simulink model "test_com_PowerLimitation_adaptTorquePart"  (R2017a)
settings: Solver=FixedStepDiscrete  StartTime=0.0  StopTime=160  RelTol=1e-3
libraries: simulink x1
settings Model: Creator=gt_testing  LastModifiedBy=rieth

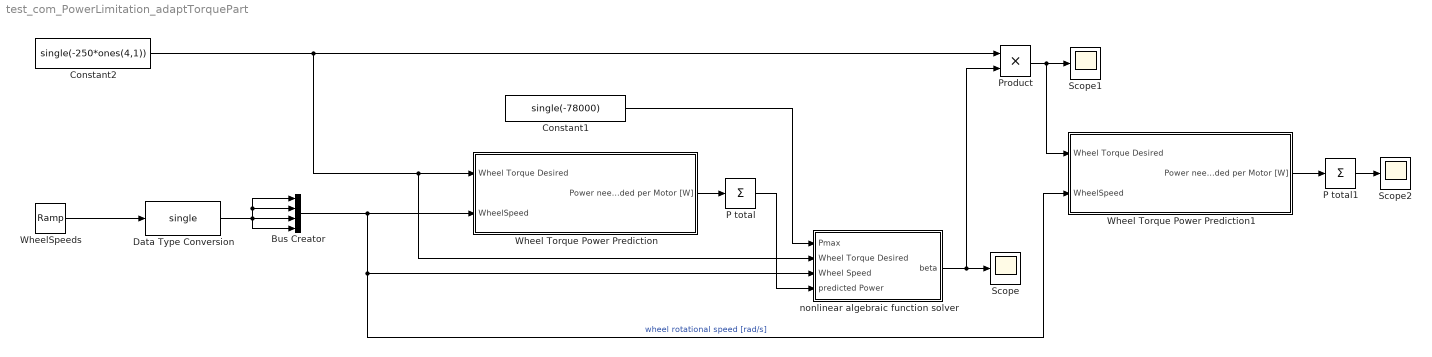
== system test_com_PowerLimitation_adaptTorquePart ==
  Bus Creator : BusCreator  Inputs=4
  Constant1 : Constant  Value=single(-78000)
  Constant2 : Constant  Value=single(-250*ones(4,1))  SampleTime=0.001
  Data Type Conversion : DataTypeConversion  OutDataTypeStr=single
  P total : Sum  Inputs=+
  P total1 : Sum  Inputs=+
  Product : Product
  Scope : Scope
  Scope1 : Scope
  Scope2 : Scope
  Wheel Torque Power Prediction : Subsystem
  Wheel Torque Power Prediction1 : Subsystem
  WheelSpeeds : simulink/Sources/Ramp  slope=-1  start=1  X0=151
  nonlinear algebraic function solver : Subsystem
  wires:
  nonlinear algebraic function solver/1(beta) -> Scope/1, Product/2
  Wheel Torque Power Prediction/1(Power needed per Motor [W]) -> P total/1
  P total/1 -> nonlinear algebraic function solver/4(predicted Power)
  Constant2/1 -> nonlinear algebraic function solver/2(Wheel Torque Desired), Wheel Torque Power Prediction/1(Wheel Torque Desired), Product/1
  Constant1/1 -> nonlinear algebraic function solver/1(Pmax)
  Bus Creator/1 -> nonlinear algebraic function solver/3(Wheel Speed), Wheel Torque Power Prediction1/2(WheelSpeed), Wheel Torque Power Prediction/2(WheelSpeed)  "wheel rotational speed [rad/s]"
  WheelSpeeds/1 -> Data Type Conversion/1
  Data Type Conversion/1 -> Bus Creator/2, Bus Creator/1, Bus Creator/4, Bus Creator/3
  Product/1 -> Scope1/1, Wheel Torque Power Prediction1/1(Wheel Torque Desired)
  Wheel Torque Power Prediction1/1(Power needed per Motor [W]) -> P total1/1
  P total1/1 -> Scope2/1

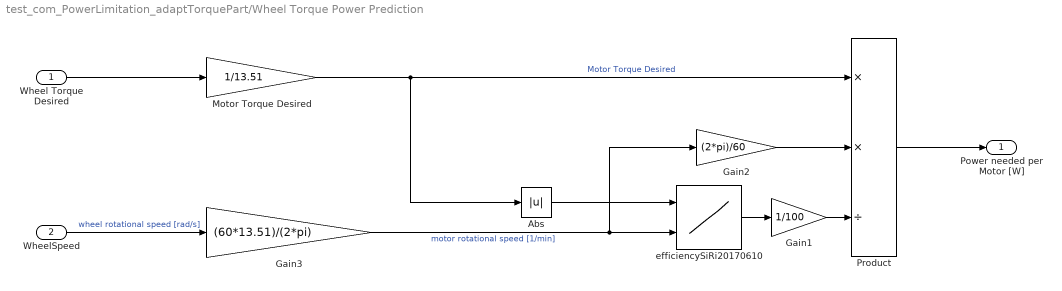
== system test_com_PowerLimitation_adaptTorquePart/Wheel Torque Power Prediction ==
  Wheel Torque Desired : Inport
  WheelSpeed : Inport  Port=2
  Abs : Abs
  Gain1 : Gain  Gain=1/100
  Gain2 : Gain  Gain=(2*pi)/60
  Gain3 : Gain  Gain=(60*13.51)/(2*pi)
  Motor Torque Desired : Gain  Gain=1/13.51
  Product : Product  Inputs=**/
  efficiencySiRi20170610 : Lookup_n-D  BreakpointsForDimension1=single([1,3.2,3.9,8.7,10,11.3,16.2,20.3,24,26.9,28.3]);  BreakpointsForDimension2=single([48,1960,3950,5880,7870,9840,11780,13740,14720,15710,17690,19640]);  Table="single( reshape( [94 93 92 91 90 90 90 90 90 90 90 90; 99.36774129\t90.61029352\t90.48980391\t90.9585099\t91.97303205\t86.66621940\t86.45154548\t89.45556778\t93.49708755\t90.20622767\t96.32187851\t93.77483204; 31.27753348\t89.58805789\t90.35051471\t91.0088400\t91.34257504\t92.79112863\t93.43970070\t92.86254617\t95.49044846\t91.88713991\t92.09660288\t99.38740423; 31.22057366\t88.54516887\t91.41259271\t91.9339048\t92.80185490\t93.37850287\t93.37968650\t93.43660779\t95.56974312\t93.62737163\t98.23400855\t97.68028598;  19.06082130\t88.16649558\t92.11595977\t92.90571858\t94.06474181\t93.59829873\t93.68368928\t93.99821230\t94.48495482\t93.64934183\t97.64599471\t99.79304925; 22.65493310\t85.04354735\t90.63432599\t90.89186387\t93.01206035\t92.42222619\t93.04151248\t93.12674620\t94.62498470\t93.19873407\t97.48235007\t99.63288088; 14.35381991\t81.97479573\t88.38188275\t90.58879348\t91.42237266\t91.86404458\t91.96724861\t92.60660720\t93.61744476\t92.73660389\t96.28617258\t97.91800590; 9.871996419\t75.78855723\t84.58478190\t87.19329262\t89.29452440\t90.10911954\t88.99885889\t91.24022984\t92.50845489\t92.30525632\t92.70068550\t95.95176799; 7.166365164\t66.33041277\t78.12603510\t81.72006745\t85.16747699\t86.66493509\t87.05734065\t89.50257798\t89.70411810\t90.50722583 90.50722583 90.50722583; 5.521446362\t64.00758121\t75.81765563\t81.30737314\t85.24988669\t87.40396493 87.40396493 87.40396493 87.40396493 87.40396493 87.40396493 87.40396493; 4.758428457\t61.91902319\t74.24685691\t80.55482871\t83.61528364\t85.08425625 85.08425625 85.08425625 85.08425625 85.08425625 85.08425625 85.08425625], 11, 12 ) );"  InternalRulePriority=Speed  RndMeth=Simplest  InputSameDT=on
  Power needed per Motor [W] : Outport  OutDataTypeStr=single
  wires:
  Wheel Torque Desired/1 -> Motor Torque Desired/1
  Motor Torque Desired/1 -> Product/1, Abs/1  "Motor Torque Desired"
  Product/1 -> Power needed per Motor [W]/1
  Abs/1 -> efficiencySiRi20170610/1
  Gain1/1 -> Product/3
  efficiencySiRi20170610/1 -> Gain1/1
  WheelSpeed/1 -> Gain3/1  "wheel rotational speed [rad/s]"
  Gain3/1 -> Gain2/1, efficiencySiRi20170610/2  "motor rotational speed [1/min]"
  Gain2/1 -> Product/2

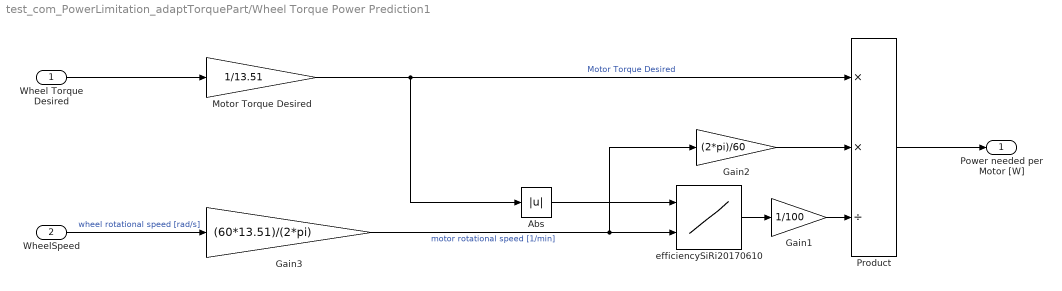
== system test_com_PowerLimitation_adaptTorquePart/Wheel Torque Power Prediction1 ==
  Wheel Torque Desired : Inport
  WheelSpeed : Inport  Port=2
  Abs : Abs
  Gain1 : Gain  Gain=1/100
  Gain2 : Gain  Gain=(2*pi)/60
  Gain3 : Gain  Gain=(60*13.51)/(2*pi)
  Motor Torque Desired : Gain  Gain=1/13.51
  Product : Product  Inputs=**/
  efficiencySiRi20170610 : Lookup_n-D  BreakpointsForDimension1=single([1,3.2,3.9,8.7,10,11.3,16.2,20.3,24,26.9,28.3]);  BreakpointsForDimension2=single([48,1960,3950,5880,7870,9840,11780,13740,14720,15710,17690,19640]);  Table="single( reshape( [94 93 92 91 90 90 90 90 90 90 90 90; 99.36774129\t90.61029352\t90.48980391\t90.9585099\t91.97303205\t86.66621940\t86.45154548\t89.45556778\t93.49708755\t90.20622767\t96.32187851\t93.77483204; 31.27753348\t89.58805789\t90.35051471\t91.0088400\t91.34257504\t92.79112863\t93.43970070\t92.86254617\t95.49044846\t91.88713991\t92.09660288\t99.38740423; 31.22057366\t88.54516887\t91.41259271\t91.9339048\t92.80185490\t93.37850287\t93.37968650\t93.43660779\t95.56974312\t93.62737163\t98.23400855\t97.68028598;  19.06082130\t88.16649558\t92.11595977\t92.90571858\t94.06474181\t93.59829873\t93.68368928\t93.99821230\t94.48495482\t93.64934183\t97.64599471\t99.79304925; 22.65493310\t85.04354735\t90.63432599\t90.89186387\t93.01206035\t92.42222619\t93.04151248\t93.12674620\t94.62498470\t93.19873407\t97.48235007\t99.63288088; 14.35381991\t81.97479573\t88.38188275\t90.58879348\t91.42237266\t91.86404458\t91.96724861\t92.60660720\t93.61744476\t92.73660389\t96.28617258\t97.91800590; 9.871996419\t75.78855723\t84.58478190\t87.19329262\t89.29452440\t90.10911954\t88.99885889\t91.24022984\t92.50845489\t92.30525632\t92.70068550\t95.95176799; 7.166365164\t66.33041277\t78.12603510\t81.72006745\t85.16747699\t86.66493509\t87.05734065\t89.50257798\t89.70411810\t90.50722583 90.50722583 90.50722583; 5.521446362\t64.00758121\t75.81765563\t81.30737314\t85.24988669\t87.40396493 87.40396493 87.40396493 87.40396493 87.40396493 87.40396493 87.40396493; 4.758428457\t61.91902319\t74.24685691\t80.55482871\t83.61528364\t85.08425625 85.08425625 85.08425625 85.08425625 85.08425625 85.08425625 85.08425625], 11, 12 ) );"  InternalRulePriority=Speed  RndMeth=Simplest  InputSameDT=on
  Power needed per Motor [W] : Outport  OutDataTypeStr=single
  wires:
  Gain2/1 -> Product/2
  Gain3/1 -> efficiencySiRi20170610/2, Gain2/1  "motor rotational speed [1/min]"
  WheelSpeed/1 -> Gain3/1  "wheel rotational speed [rad/s]"
  efficiencySiRi20170610/1 -> Gain1/1
  Gain1/1 -> Product/3
  Abs/1 -> efficiencySiRi20170610/1
  Product/1 -> Power needed per Motor [W]/1
  Motor Torque Desired/1 -> Abs/1, Product/1  "Motor Torque Desired"
  Wheel Torque Desired/1 -> Motor Torque Desired/1

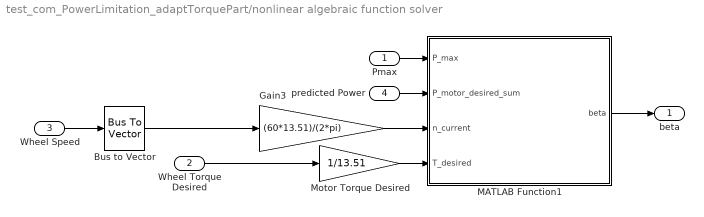
== system test_com_PowerLimitation_adaptTorquePart/nonlinear algebraic function solver ==
  Pmax : Inport
  Wheel Torque Desired : Inport  Port=2
  Wheel Speed : Inport  Port=3
  predicted Power : Inport  Port=4
  Bus to Vector : BusToVector
  Gain3 : Gain  Gain=(60*13.51)/(2*pi)
  MATLAB Function1 : MATLAB Function  TreatAsAtomicUnit=on
  Motor Torque Desired : Gain  Gain=1/13.51
  beta : Outport
  wires:
  MATLAB Function1/1(beta) -> beta/1
  Pmax/1 -> MATLAB Function1/1(P_max)
  Wheel Torque Desired/1 -> Motor Torque Desired/1
  Wheel Speed/1 -> Bus to Vector/1
  Motor Torque Desired/1 -> MATLAB Function1/4(T_desired)
  Bus to Vector/1 -> Gain3/1
  Gain3/1 -> MATLAB Function1/3(n_current)
  predicted Power/1 -> MATLAB Function1/2(P_motor_desired_sum)

== matlab function test_com_PowerLimitation_adaptTorquePart/nonlinear algebraic function solver/MATLAB Function1 ==
  data: P_max input single size=1; P_motor_desired_sum input single size=[1 1]; n_current input single size=[4,1]; T_desired input; beta output single size=1
function beta  = adaptTorque( P_max, P_motor_desired_sum, n_current,T_desired)

P_max = abs(P_max);
P_motor_desired_sum = abs(P_motor_desired_sum);
T_desired = abs(T_desired);

efficiency = zeros(4,1);
% efficiency_desired = zeros(4,1);

efficiency_complete = single( reshape( [94 93 92 91 90 90 90 90 90 90 90 90; ... 
                                        99.36774129	90.61029352	90.48980391	90.9585099	91.97303205	86.66621940	86.45154548	89.45556778	93.49708755	90.20622767	96.32187851	93.77483204; ...
                                        31.27753348	89.58805789	90.35051471	91.0088400	91.34257504	92.79112863	93.43970070	92.86254617	95.49044846	91.88713991	92.09660288	99.38740423; ...
                                        31.22057366	88.54516887	91.41259271	91.9339048	92.80185490	93.37850287	93.37968650	93.43660779	95.56974312	93.62737163	98.23400855	97.68028598; ...
                                        19.06082130	88.16649558	92.11595977	92.90571858	94.06474181	93.59829873	93.68368928	93.99821230	94.48495482	93.64934183	97.64599471	99.79304925; ...
                                        22.65493310	85.04354735	90.63432599	90.89186387	93.01206035	92.42222619	93.04151248	93.12674620	94.62498470	93.19873407	97.48235007	99.63288088; ...
                                        14.35381991	81.97479573	88.38188275	90.58879348	91.42237266	91.86404458	91.96724861	92.60660720	93.61744476	92.73660389	96.28617258	97.91800590; ...
                                        9.871996419	75.78855723	84.58478190	87.19329262	89.29452440	90.10911954	88.99885889	91.24022984	92.50845489	92.30525632	92.70068550	95.95176799; ...
                                        7.166365164	66.33041277	78.12603510	81.72006745	85.16747699	86.66493509	87.05734065	89.50257798	89.70411810	90.50722583 90.50722583 90.50722583; ...
                                        5.521446362	64.00758121	75.81765563	81.30737314	85.24988669	87.40396493 87.40396493 87.40396493 87.40396493 87.40396493 87.40396493 87.40396493; ...
                                        4.758428457	61.91902319	74.24685691	80.55482871	83.61528364	85.08425625 85.08425625 85.08425625 85.08425625 85.08425625 85.08425625 85.08425625], 11, 12 ) );
                         
T_complete = single([1,3.2,3.9,8.7,10,11.3,16.2,20.3,24,26.9,28.3]);
n_complete = single([48,1960,3950,5880,7870,9840,11780,13740,14720,15710,17690,19640]); 

n_current_radps = 2*pi/60 * n_current; %n_current in umdrehungen pro minute, umrechnung in rad pro sekunde 

% %Abfangen von out-of-range Werten
% for i = 1:4
%     if abs(T_desired(i)) > 28.3 
%         T_desired(i) = sign(T_desired(i))*single(28.3);
%     elseif T_desired(i) < 1
%         T_desired(i) = sign(T_desired(i))*single(1);
%     end
% end
% 
% efficiency_desired(1) = diag( interpn( T_complete, n_complete, efficiency_complete, abs(T_desired(1)), n_current(1), 'linear' ) ) / 100; %percentage
% efficiency_desired(2) = diag( interpn( T_complete, n_complete, efficiency_complete, abs(T_desired(2)), n_current(2), 'linear' ) ) / 100; %percentage
% efficiency_desired(3) = diag( interpn( T_complete, n_complete, efficiency_complete, abs(T_desired(3)), n_current(3), 'linear' ) ) / 100; %percentage
% efficiency_desired(4) = diag( interpn( T_complete, n_complete, efficiency_complete, abs(T_desired(4)), n_current(4), 'linear' ) ) / 100; %percentage
% 
% P_motor_desired_fl = T_desired(1)*n_current_radps(1)/efficiency_desired(1);
% P_motor_desired_fr = T_desired(2)*n_current_radps(2)/efficiency_desired(2);
% P_motor_desired_rl = T_desired(3)*n_current_radps(3)/efficiency_desired(3);
% P_motor_desired_rr = T_desired(4)*n_current_radps(4)/efficiency_desired(4);
% 
% P_motor_desired_sum = P_motor_desired_fl + P_motor_desired_fr + P_motor_desired_rl + P_motor_desired_rr;


% 
% if x < 0
%     x = single(0);
% elseif x > 1
%     x = single(1);
% end

T_adapted_old = T_desired + 1;
efficiency_old = single( zeros( 4, 1 ) );
T_adapted = T_desired;
P_Whatever = single( zeros( 4, 1 ) );
P_motor_adap_sum = P_motor_desired_sum;
condAdaptionCalculation = P_motor_adap_sum - P_max;

if condAdaptionCalculation > 0
    x = P_max/P_motor_desired_sum;
else
	x = single(1);
end

while condAdaptionCalculation > 0
    
    %Abfangen von out-of-range Werten
    for i = 1:4
        if abs(T_adapted(i)) > 28.3 
            T_adapted(i) = single(28.3);
        elseif T_adapted(i) < 1
            T_adapted(i) = single(1);
        end
    end
    
    % Berechnen des Wirkungsgrades mittels angepasstem Moment
    efficiency(1) = diag( interpn( T_complete, n_complete, efficiency_complete, T_adapted(1), n_current(1), 'linear' ) ) / 100; %percentage
    efficiency(2) = diag( interpn( T_complete, n_complete, efficiency_complete, T_adapted(2), n_current(2), 'linear' ) ) / 100; %percentage
    efficiency(3) = diag( interpn( T_complete, n_complete, efficiency_complete, T_adapted(3), n_current(3), 'linear' ) ) / 100; %percentage
    efficiency(4) = diag( interpn( T_complete, n_complete, efficiency_complete, T_adapted(4), n_current(4), 'linear' ) ) / 100; %percentage
        
    % Ableiten der Effizienz nach Korrekturfaktor
    DEfficiency_fl = ( efficiency(1) - efficiency_old(1) )./( T_adapted(1) - T_adapted_old(1) );
    DEfficiency_fr = ( efficiency(2) - efficiency_old(2) )./( T_adapted(2) - T_adapted_old(2) );
    DEfficiency_rl = ( efficiency(3) - efficiency_old(3) )./( T_adapted(3) - T_adapted_old(3) );
    DEfficiency_rr = ( efficiency(4) - efficiency_old(4) )./( T_adapted(4) - T_adapted_old(4) );
    DEfficiency = [DEfficiency_fl;DEfficiency_fr;DEfficiency_rl;DEfficiency_rr];
    
    % induced power 
    P_motor_ind_fl = T_adapted_old(1)*n_current_radps(1)/efficiency(1); 
    P_motor_ind_fr = T_adapted_old(2)*n_current_radps(2)/efficiency(2);
    P_motor_ind_rl = T_adapted_old(3)*n_current_radps(3)/efficiency(3);
    P_motor_ind_rr = T_adapted_old(4)*n_current_radps(4)/efficiency(4);    
    P_motor_ind = [P_motor_ind_fl;P_motor_ind_fr;P_motor_ind_rl;P_motor_ind_rr]; 
         
    % adapted induced power
    P_motor_adap_fl = T_adapted(1)*n_current_radps(1)/efficiency(1); 
    P_motor_adap_fr = T_adapted(2)*n_current_radps(2)/efficiency(2);
    P_motor_adap_rl = T_adapted(3)*n_current_radps(3)/efficiency(3);
    P_motor_adap_rr = T_adapted(4)*n_current_radps(4)/efficiency(4);    
    P_motor_adap_sum = P_motor_adap_fl + P_motor_adap_fr + P_motor_adap_rl + P_motor_adap_rr;
    
    P_nonlin_function = P_motor_adap_sum - P_max;    
    
    P_Whatever(1) = T_adapted(1)^2*n_current_radps(1)*DEfficiency(1)/efficiency(1)^2;
    P_Whatever(2) = T_adapted(2)^2*n_current_radps(2)*DEfficiency(2)/efficiency(2)^2;
    P_Whatever(3) = T_adapted(3)^2*n_current_radps(3)*DEfficiency(3)/efficiency(3)^2;
    P_Whatever(4) = T_adapted(4)^2*n_current_radps(4)*DEfficiency(4)/efficiency(4)^2;
    
    P_diff_sum = sum( P_motor_ind - P_Whatever );
    
    efficiency_old = single(efficiency);
    T_adapted_old = T_adapted;

    if P_diff_sum == 0 || isnan(P_diff_sum)
        P_diff_sum = single(1e5);
    end

    x = x - P_nonlin_function / P_diff_sum;
    T_adapted = x * T_adapted;
    if x < 0
        x = single(0);
    elseif x > 1
        x = single(1);
	end
	condAdaptionCalculation = P_motor_adap_sum - P_max;
end
if x < 0
    beta = single(0);
elseif x > 1
    beta = single(1);
else
    beta = x;
end
